simulink model "Worked_Example_7_3"  (R2024b)
settings: Solver=VariableStepAuto  StartTime=0.0  StopTime=15  RelTol=1e-3
settings Model: Creator=GH-X-ST  LastModifiedBy=GH-X-ST

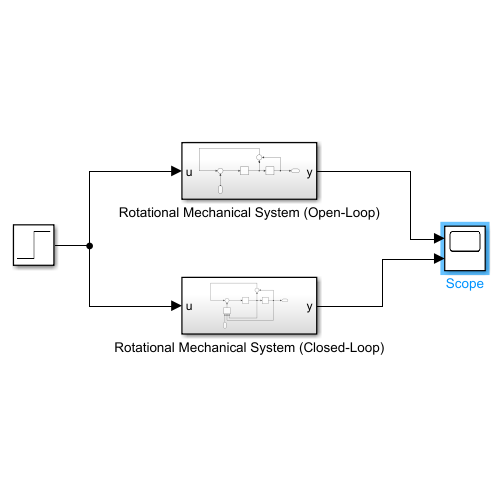
[thumbnail: Simulink's stored preview of the top-level diagram]
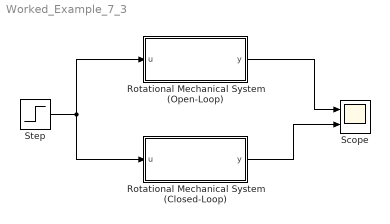
== system Worked_Example_7_3 ==
  Rotational Mechanical System (Closed-Loop) : Subsystem
  Rotational Mechanical System (Open-Loop) : Subsystem
  Scope : Scope  NumInputPorts=2
  Step : Step  SampleTime=0
  wires:
  Rotational Mechanical System (Open-Loop)/1(y) -> Scope/1
  Step/1 -> Rotational Mechanical System (Open-Loop)/1(u), Rotational Mechanical System (Closed-Loop)/1(u)
  Rotational Mechanical System (Closed-Loop)/1(y) -> Scope/2

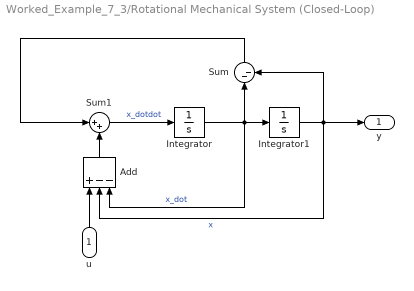
== system Worked_Example_7_3/Rotational Mechanical System (Closed-Loop) ==
  u : Inport
  Add : Sum  Inputs=+--
  Integrator : Integrator
  Integrator1 : Integrator
  Sum : Sum  Inputs=|--
  Sum1 : Sum  Inputs=|++
  y : Outport
  wires:
  Integrator/1 -> Add/3, Sum/1, Integrator1/1  "x_dot"
  Integrator1/1 -> Add/2, y/1, Sum/2  "x"
  Sum/1 -> Sum1/1
  Sum1/1 -> Integrator/1  "x_dotdot"
  u/1 -> Add/1
  Add/1 -> Sum1/2

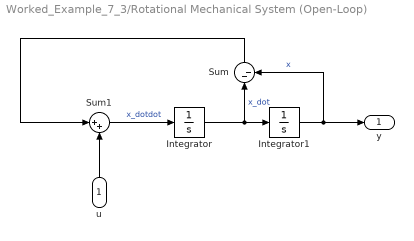
== system Worked_Example_7_3/Rotational Mechanical System (Open-Loop) ==
  u : Inport
  Integrator : Integrator
  Integrator1 : Integrator
  Sum : Sum  Inputs=|--
  Sum1 : Sum  Inputs=|++
  y : Outport
  wires:
  Integrator/1 -> Integrator1/1, Sum/1  "x_dot"
  Integrator1/1 -> y/1, Sum/2  "x"
  Sum/1 -> Sum1/1
  u/1 -> Sum1/2
  Sum1/1 -> Integrator/1  "x_dotdot"
